simulink model "solar_grid_powered_EV_Battery_Charging_station"  (R2020a)
settings: Solver=VariableStepAuto  StartTime=0.0  StopTime=1  RelTol=1e-3
undefined symbols (not defined in the file): Ion, Lithium
libraries: powerlib x68, simulink x10, powerlib_meascontrol x4, electricdrivelib x1, re_lib x1
(part 1 of 2)
settings Model: Creator=sunil  LastModifiedBy=sunil

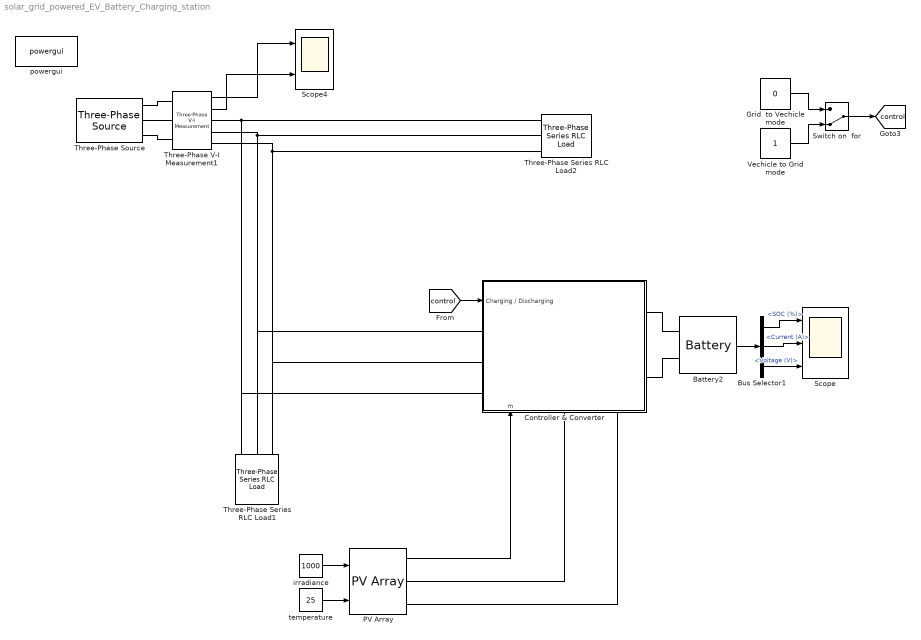
== system solar_grid_powered_EV_Battery_Charging_station ==
  Battery2 : electricdrivelib/Extra Sources/Battery  BatType=Lithium-Ion  ShowTempParam=off  ThermalPreset=no  ShowAgeParam=off  NomV=250  NomQ=300  SOC=80  Batt_Tr=30  PresetModel=on  MaxQ=300  MinV=187.5  FullV=290.9968  Dis_rate=130.4348  R=0.0083333  Normal_OP=271.3043  expZone="[270.0965      14.73913]"  current=[6.5 13 32.5]  Units=Time  Tci=20  NomT=20  T2=-30  MaxQ2=4.8  FullV2=7.1  Normal_OP2=5.655  expZone2="[6.58           1]"  Rca=0.6  ti=2000  Dp=0  Neq0=0  Tsim=1e6  Ta1=25  Qeol=5.4*0.9  Reol=0.013333*1.2  Char_age=[2.3478, 3]  Dis_age=[2.3478, 10]  N1=1500  N2=10500  N3=1000  N4=1400  Ta2=45  N5=950
  Bus Selector1 : BusSelector  OutputSignals=SOC (%),Current (A),Voltage (V)
  Controller & Converter : Subsystem
      settings: PortSchema="{\"entries\":[{\"content\":{\"sides\":[{\"content\":{\"connectorIds\":[\"In1\",\"LConn1\",\"LConn2\",\"LConn3\"]},\"type\":\"ConnectorPlacement.EquallySpacedRectSide\",\"uuid\":\"3304ff68-ecae-43f2-8867-5e121d5d8c98\"},{\"content\":{\"connectorIds\":[\"RConn1\",\"RConn2\"],\"side\":\"RIGHT\"},\"type\":\"ConnectorPlacement.EquallySpacedRectSide\",\"uuid\":\"3bd92547-fde4-4d16-9531-59e3d4d1a2fd\"},{\"content\":{\"connectorIds\":[],\"side\":\"TOP\"},\"type\":\"ConnectorPlacement.EquallySpacedRectSide\",\"uuid\":\"a99ca367-b74d-41f6-b4fc-d39809732728\"},{\"content\":{\"connectorIds\":[\"In2\",\"RConn3\",\"RConn4\"],\"side\":\"BOTTOM\"},\"type\":\"ConnectorPlacement.EquallySpacedRectSide\",\"uuid\":\"df3368a7-37c5-4fdd-8e4a-104a2c6a0ba1\"}]},\"type\":\"ConnectorPlacement.EquallySpacedConnector\",\"uuid\":\"9d0b0e84-d3bf-47a7-98c1-fe37fca38536\"}],\"packageUris\":[\"http://schema.mathworks.com/mf0/Connector/19700101\"],\"version\":\"1.0\"}"
  Grid  to Vechicle mode : Constant  Value=0  VectorParams1D=off  SampleTime=-1
  PV Array : re_lib/Solar/PV Array  Npar=10  Nser=7  PlotType=array @ 25 deg.C & specified irradiances  S_vec="[ 1000  500  100 ]"  Temp_C_vec="[ 45 25  ]"  ModuleName=User-defined  PlotWhenSelected=off  Pm=390.173  Ncell=72  Voc=48.85  Isc=10  Vm=40.1  Im=9.73  beta_Voc_pc=-0.37  alpha_Isc_pc=0.05  beta_Voc=-0.18075  alpha_Isc=0.005  IL=10.1848  I0=4.7391e-10  nI=1.1101  Rsh=3123.3273  Rs=0.27721  RobustModel=off  RobustCellTemperature=25  BAL=on  Tc=1e-6  Tfilter=5e-5
  Scope : Scope  NumInputPorts=3
  Scope4 : Scope  NumInputPorts=2
  "Switch on  for " : ManualSwitch  CurrentSetting=0
  Three-Phase Series RLC Load1 : powerlib/Elements/Three-Phase Series RLC Load  LConnTagsString=A|B|C  Configuration=Y (grounded)  NominalVoltage=415  Vabc=[1e3 1e3 1e3]  Vabcp=[1e3 1e3 1e3]  NominalFrequency=50  UnbalancedPower=off  ActivePower=1e3  InductivePower=0  CapacitivePower=0  Pabc=[10e3 9e3 11e3]  QLabc=[100 90 110]  QCabc=[100 90 110]  Pabcp=[10e3 9e3 11e3]  QLabcp=[100 90 110]  QCabcp=[100 90 110]  Measurements=None  LoadType=constant Z
  Three-Phase Series RLC Load2 : powerlib/Elements/Three-Phase Series RLC Load  LConnTagsString=A|B|C  Configuration=Y (grounded)  NominalVoltage=415  Vabc=[1e3 1e3 1e3]  Vabcp=[1e3 1e3 1e3]  NominalFrequency=50  UnbalancedPower=off  ActivePower=1e-3  InductivePower=0  CapacitivePower=0  Pabc=[10e3 9e3 11e3]  QLabc=[100 90 110]  QCabc=[100 90 110]  Pabcp=[10e3 9e3 11e3]  QLabcp=[100 90 110]  QCabcp=[100 90 110]  Measurements=None  LoadType=constant Z
  Three-Phase V-I Measurement1 : powerlib/Measurements/Three-Phase V-I Measurement  VoltageMeasurement=phase-to-phase  SetLabelV=off  LabelV=Vabc  Vpu=off  VpuLL=off  CurrentMeasurement=yes  SetLabelI=off  LabelI=Iabc  Ipu=off  Pbase=100e6  Vbase=500e3  OutputType=Complex  PhasorSimulation=off  PSBequivalent=0
  Three-Phase Source : powerlib/Electrical Sources/Three-Phase Source  InternalConnection=Yg  VoltagePhases=off  Voltage=415  PhaseAngle=0  Voltage_phases=[25e3 25e3 25e3]/sqrt(3)  PhaseAngles_phases=[0 -120 +120]  Frequency=50  NonIdealSource=on  SpecifyImpedance=off  Resistance=1e-6  Inductance=1e-6  ShortCircuitLevel=100e6  BaseVoltage=415  XRratio=7  BusType=swing  Pref=10e3  Qref=0  Prefabc=[10e3, 10e3, 10e3]  Qrefabc=[0, 0, 0]  Qmin=-inf  Qmax=inf
  Vechicle to Grid mode : Constant  VectorParams1D=off  SampleTime=-1
  irradiance : Constant  Value=1000
  powergui : powerlib/powergui  Priority=1  SimulationMode=Discrete  SampleTime=5e-6  frequency=60  Iterations=50  frequencyindice=0  Pbase=100e6  ErrMax=1e-4  UnitsV=kV  UnitsW=MW  buscounter=0  FunctionMessages=off  echomessages=off  EnableUseOfTLC=off  CurrentSourceSwitches=off  DisableSnubberDevices=off  DisableRonSwitches=off  DisableVfSwitches=off  DisplayEquations=off  AutomaticDiscreteSolvers=off  SolverType=Tustin/Backward Euler (TBE)  Interpol=off  ExternalGateDelay=off  methode=off  Ts=100  x0status=blocks  SPID=on  SwTol=0  HookPort=off  NonlinearTolerance=1e-4  nMaxIteration=100  ContinueOnMaxIteration=off  RestoreLinks=warning  ResistiveCurrentMeasurement=off  Frange=[0:2:500]  Ylog=off  Xlog=on  ShowGrid=off  save=off  variable=ZData  structure=0  ZoomFFT=off  StartTime=0.0  cycles=1  DisplayStyle=1  fundamental=60  FreqAxis=off  MaxFrequency=1000  frequencyindicesteady=1  RmsSteady=1  display=off
  temperature : Constant  Value=25
  tag scope: control=global
  wires:
  Bus Selector1/2 -> Scope/2  "<Current (A)>"
  Grid  to Vechicle mode/1 -> "Switch on  for "/1
  [control] -> Controller & Converter/1(Charging / Discharging)
  Bus Selector1/3 -> Scope/3  "<Voltage (V)>"
  Vechicle to Grid mode/1 -> "Switch on  for "/2
  Bus Selector1/1 -> Scope/1  "<SOC (%)>"
  Three-Phase V-I Measurement1/2 -> Scope4/2
  Battery2/1 -> Bus Selector1/1
  temperature/1 -> PV Array/2
  Three-Phase V-I Measurement1/1 -> Scope4/1
  "Switch on  for "/1 -> [control]
  PV Array/1 -> Controller & Converter/2(m)
  irradiance/1 -> PV Array/1
  connections:
  Three-Phase Series RLC Load2/LConn2 -- Three-Phase Series RLC Load1/LConn2 -- Controller & Converter/LConn1 -- Three-Phase V-I Measurement1/RConn2
  Three-Phase Series RLC Load2/LConn3 -- Three-Phase V-I Measurement1/RConn3 -- Three-Phase Series RLC Load1/LConn3 -- Controller & Converter/LConn2
  Three-Phase Series RLC Load2/LConn1 -- Three-Phase Series RLC Load1/LConn1 -- Controller & Converter/LConn3 -- Three-Phase V-I Measurement1/RConn1
  Battery2/LConn1 -- Controller & Converter/RConn1
  Three-Phase V-I Measurement1/LConn3 -- Three-Phase Source/RConn3
  PV Array/RConn2 -- Controller & Converter/RConn4
  Three-Phase V-I Measurement1/LConn2 -- Three-Phase Source/RConn2
  Battery2/LConn2 -- Controller & Converter/RConn2
  Three-Phase V-I Measurement1/LConn1 -- Three-Phase Source/RConn1
  PV Array/RConn1 -- Controller & Converter/RConn3

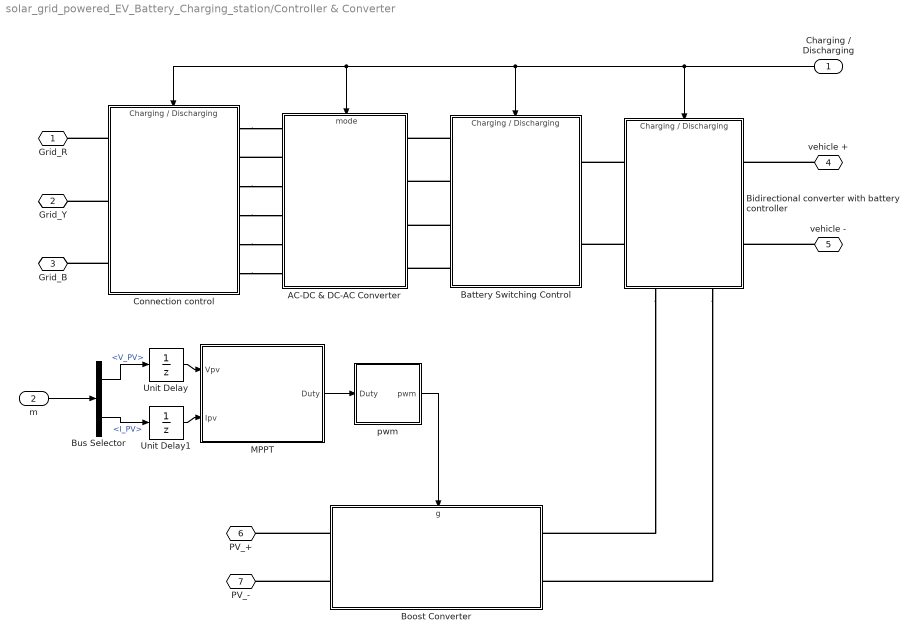
== system solar_grid_powered_EV_Battery_Charging_station/Controller & Converter ==
  Charging / Discharging : Inport
  m : Inport  Port=2
  AC-DC & DC-AC Converter : Subsystem
      settings: PortSchema="{\"entries\":[{\"content\":{\"sides\":[{\"content\":{\"connectorIds\":[\"LConn1\",\"LConn2\",\"LConn3\",\"LConn4\",\"LConn5\",\"LConn6\"]},\"type\":\"ConnectorPlacement.EquallySpacedRectSide\",\"uuid\":\"fb71d267-2bb0-4139-94a5-dc54601bb02f\"},{\"content\":{\"connectorIds\":[\"RConn1\",\"RConn2\",\"RConn3\",\"RConn4\"],\"side\":\"RIGHT\"},\"type\":\"ConnectorPlacement.EquallySpacedRectSide\",\"uuid\":\"de844200-b1ec-408d-a180-7fb4681b7df4\"},{\"content\":{\"connectorIds\":[\"In1\"],\"side\":\"TOP\"},\"type\":\"ConnectorPlacement.EquallySpacedRectSide\",\"uuid\":\"9cac342e-4efb-4690-aa53-18569bafd674\"}]},\"type\":\"ConnectorPlacement.EquallySpacedConnector\",\"uuid\":\"f9655260-9e6f-4e0e-a67b-e2fec888fb30\"}],\"packageUris\":[\"http://schema.mathworks.com/mf0/Connector/19700101\"],\"version\":\"1.0\"}"
  Battery Switching Control : Subsystem
      settings: PortSchema="{\"entries\":[{\"content\":{\"sides\":[{\"content\":{\"connectorIds\":[\"LConn1\",\"LConn2\",\"LConn3\",\"LConn4\"]},\"type\":\"ConnectorPlacement.EquallySpacedRectSide\",\"uuid\":\"d80df2a9-ec6b-4c90-bb66-bcdaf5f87525\"},{\"content\":{\"connectorIds\":[\"RConn1\",\"RConn2\"],\"side\":\"RIGHT\"},\"type\":\"ConnectorPlacement.EquallySpacedRectSide\",\"uuid\":\"2e5caa84-3c0f-4e6e-a9f1-36c129bda481\"},{\"content\":{\"connectorIds\":[\"In1\"],\"side\":\"TOP\"},\"type\":\"ConnectorPlacement.EquallySpacedRectSide\",\"uuid\":\"9ad9ed80-d46f-43fc-be26-7456a6f75322\"},{\"content\":{\"connectorIds\":[],\"side\":\"BOTTOM\"},\"type\":\"ConnectorPlacement.EquallySpacedRectSide\",\"uuid\":\"36c54608-1582-475c-a859-dff20a425875\"}]},\"type\":\"ConnectorPlacement.EquallySpacedConnector\",\"uuid\":\"78778afb-b988-47e6-8bc2-703e283fa2d4\"}],\"packageUris\":[\"http://schema.mathworks.com/mf0/Connector/19700101\"],\"version\":\"1.0\"}"
  Bidirectional converter with battery controller : Subsystem
      settings: PortSchema="{\"entries\":[{\"content\":{\"sides\":[{\"content\":{\"connectorIds\":[\"LConn1\",\"LConn2\"]},\"type\":\"ConnectorPlacement.EquallySpacedRectSide\",\"uuid\":\"86880c34-88a1-4209-bf34-ac5a91279ce4\"},{\"content\":{\"connectorIds\":[\"RConn1\",\"RConn2\"],\"side\":\"RIGHT\"},\"type\":\"ConnectorPlacement.EquallySpacedRectSide\",\"uuid\":\"9dcfc645-7c2c-4fe1-9bcb-24debf25abab\"},{\"content\":{\"connectorIds\":[\"In1\"],\"side\":\"TOP\"},\"type\":\"ConnectorPlacement.EquallySpacedRectSide\",\"uuid\":\"a2f7b554-97d3-490c-a983-3514cfd45afe\"},{\"content\":{\"connectorIds\":[\"RConn3\",\"RConn4\"],\"side\":\"BOTTOM\"},\"type\":\"ConnectorPlacement.EquallySpacedRectSide\",\"uuid\":\"9f51b392-4a7b-4452-b01e-9bc26600887f\"}]},\"type\":\"ConnectorPlacement.EquallySpacedConnector\",\"uuid\":\"53695bd3-452d-4933-bbd5-5b98019d2721\"}],\"packageUris\":[\"http://schema.mathworks.com/mf0/Connector/19700101\"],\"version\":\"1.0\"}"
  Boost Converter : Subsystem
      settings: PortSchema="{\"entries\":[{\"content\":{\"sides\":[{\"content\":{\"connectorIds\":[\"LConn1\",\"LConn2\"]},\"type\":\"ConnectorPlacement.EquallySpacedRectSide\",\"uuid\":\"ba3df88f-bd8f-4585-9ccf-ee80b9ae1df7\"},{\"content\":{\"connectorIds\":[\"RConn1\",\"RConn2\"],\"side\":\"RIGHT\"},\"type\":\"ConnectorPlacement.EquallySpacedRectSide\",\"uuid\":\"07e3c8e5-cf0e-4606-afd9-e4eed787cba4\"},{\"content\":{\"connectorIds\":[\"In1\"],\"side\":\"TOP\"},\"type\":\"ConnectorPlacement.EquallySpacedRectSide\",\"uuid\":\"0b82548a-ce43-4895-b683-aaa03795dd24\"}]},\"type\":\"ConnectorPlacement.EquallySpacedConnector\",\"uuid\":\"1dcff1c7-df30-47a9-a5da-6bd033c00133\"}],\"packageUris\":[\"http://schema.mathworks.com/mf0/Connector/19700101\"],\"version\":\"1.0\"}"
  Bus Selector : BusSelector  OutputSignals=V_PV,I_PV
  Connection control : Subsystem
      settings: PortSchema="{\"entries\":[{\"content\":{\"sides\":[{\"content\":{\"connectorIds\":[\"LConn1\",\"LConn2\",\"LConn3\"]},\"type\":\"ConnectorPlacement.EquallySpacedRectSide\",\"uuid\":\"4b804f5e-ccd8-48e4-9dd4-f3e4f4f04b31\"},{\"content\":{\"connectorIds\":[\"RConn1\",\"RConn2\",\"RConn3\",\"RConn4\",\"RConn5\",\"RConn6\"],\"side\":\"RIGHT\"},\"type\":\"ConnectorPlacement.EquallySpacedRectSide\",\"uuid\":\"f88efa6c-9e5b-45b8-93e8-1425e80d8a81\"},{\"content\":{\"connectorIds\":[\"In1\"],\"side\":\"TOP\"},\"type\":\"ConnectorPlacement.EquallySpacedRectSide\",\"uuid\":\"34942438-89d1-493a-a64f-7ff1173d7d06\"}]},\"type\":\"ConnectorPlacement.EquallySpacedConnector\",\"uuid\":\"62c4ca2c-a19a-421e-ab33-e75936f0a9d2\"}],\"packageUris\":[\"http://schema.mathworks.com/mf0/Connector/19700101\"],\"version\":\"1.0\"}"
  MPPT : Subsystem
  Unit Delay : UnitDelay  SampleTime=1e-4  HasFrameUpgradeWarning=on
  Unit Delay1 : UnitDelay  SampleTime=1e-4  HasFrameUpgradeWarning=on
  pwm : Subsystem
  Grid_R : PMIOPort  Side=Left
  Grid_Y : PMIOPort  Port=2  Side=Left
  Grid_B : PMIOPort  Port=3  Side=Left
  vehicle + : PMIOPort  Port=4  Side=Right
  vehicle - : PMIOPort  Port=5  Side=Right
  PV_+ : PMIOPort  Port=6  Side=Right
  PV_- : PMIOPort  Port=7  Side=Right
  wires:
  Charging / Discharging/1 -> Battery Switching Control/1(Charging / Discharging), AC-DC & DC-AC Converter/1(mode), Connection control/1(Charging / Discharging), Bidirectional converter with battery controller/1(Charging / Discharging)
  Bus Selector/1 -> Unit Delay/1  "<V_PV>"
  Unit Delay1/1 -> MPPT/2(Ipv)
  MPPT/1(Duty) -> pwm/1(Duty)
  Bus Selector/2 -> Unit Delay1/1  "<I_PV>"
  Unit Delay/1 -> MPPT/1(Vpv)
  pwm/1(pwm) -> Boost Converter/1(g)
  m/1 -> Bus Selector/1
  connections:
  Connection control/LConn1 -- Grid_R/RConn1
  Connection control/LConn2 -- Grid_Y/RConn1
  Connection control/LConn3 -- Grid_B/RConn1
  AC-DC & DC-AC Converter/LConn2 -- Connection control/RConn2
  Connection control/RConn1 -- AC-DC & DC-AC Converter/LConn1
  Connection control/RConn3 -- AC-DC & DC-AC Converter/LConn3
  Connection control/RConn4 -- AC-DC & DC-AC Converter/LConn4
  Connection control/RConn5 -- AC-DC & DC-AC Converter/LConn5
  Connection control/RConn6 -- AC-DC & DC-AC Converter/LConn6
  vehicle +/RConn1 -- Bidirectional converter with battery controller/RConn1
  vehicle -/RConn1 -- Bidirectional converter with battery controller/RConn2
  Bidirectional converter with battery controller/LConn1 -- Battery Switching Control/RConn1
  Bidirectional converter with battery controller/LConn2 -- Battery Switching Control/RConn2
  Battery Switching Control/LConn1 -- AC-DC & DC-AC Converter/RConn1
  Battery Switching Control/LConn2 -- AC-DC & DC-AC Converter/RConn2
  Battery Switching Control/LConn3 -- AC-DC & DC-AC Converter/RConn3
  Battery Switching Control/LConn4 -- AC-DC & DC-AC Converter/RConn4
  Boost Converter/LConn1 -- PV_+/RConn1
  Boost Converter/LConn2 -- PV_-/RConn1
  Bidirectional converter with battery controller/RConn3 -- Boost Converter/RConn1
  Bidirectional converter with battery controller/RConn4 -- Boost Converter/RConn2

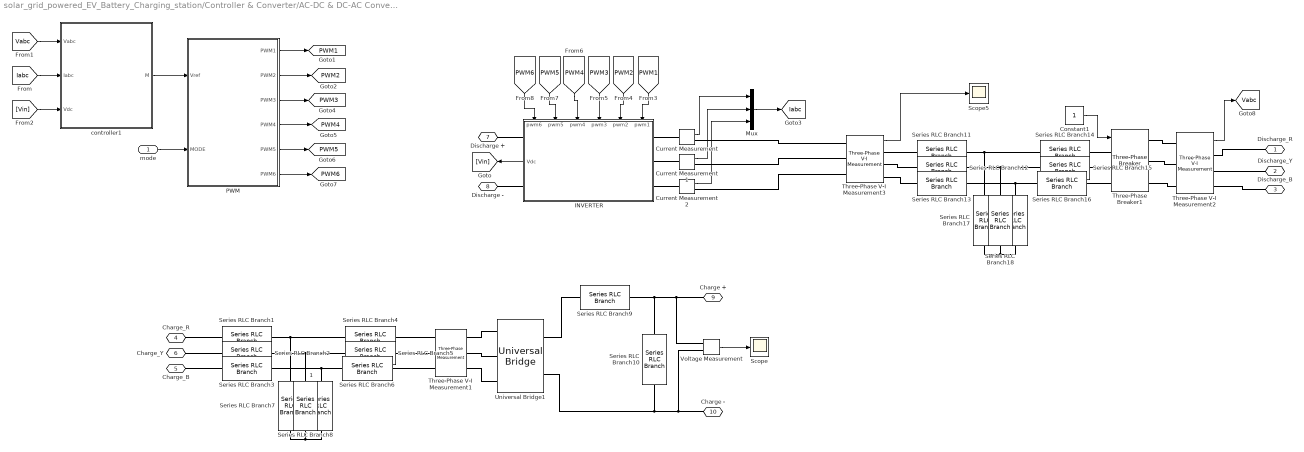
== system solar_grid_powered_EV_Battery_Charging_station/Controller & Converter/AC-DC & DC-AC Converter ==
  mode : Inport
  " " : powerlib/Elements/Series RLC Branch  LConnTagsString=__new0  RConnTagsString=__new0  BranchType=C  Resistance=1  Inductance=500e-6  SetiL0=off  InitialCurrent=0  Capacitance=100e-6  Setx0=off  InitialVoltage=0  Measurements=None
  " 1" : powerlib/Elements/Series RLC Branch  LConnTagsString=__new0  RConnTagsString=__new0  BranchType=C  Resistance=1  Inductance=500e-6  SetiL0=off  InitialCurrent=0  Capacitance=100e-6  Setx0=off  InitialVoltage=0  Measurements=None
  Constant1 : Constant
  Current Measurement : powerlib/Measurements/Current Measurement  PhasorSimulation=off  OutputType=Complex  PSBequivalent=0
  Current Measurement1 : powerlib/Measurements/Current Measurement  PhasorSimulation=off  OutputType=Complex  PSBequivalent=0
  Current Measurement2 : powerlib/Measurements/Current Measurement  PhasorSimulation=off  OutputType=Complex  PSBequivalent=0
  INVERTER : Subsystem
      settings: PortSchema="{\"entries\":[{\"content\":{\"sides\":[{\"content\":{\"connectorIds\":[\"LConn1\",\"Out1\",\"LConn2\"]},\"type\":\"ConnectorPlacement.EquallySpacedRectSide\",\"uuid\":\"c3946ff9-9688-4b39-8168-58c2573ee620\"},{\"content\":{\"connectorIds\":[\"RConn1\",\"RConn2\",\"RConn3\"],\"side\":\"RIGHT\"},\"type\":\"ConnectorPlacement.EquallySpacedRectSide\",\"uuid\":\"a5e23abb-073e-446d-99b2-4b67fe8ba86f\"},{\"content\":{\"connectorIds\":[\"In1\",\"In2\",\"In3\",\"In4\",\"In5\",\"In6\"],\"side\":\"TOP\"},\"type\":\"ConnectorPlacement.EquallySpacedRectSide\",\"uuid\":\"619d3410-10ed-4be1-83e0-3a782e5fb67e\"},{\"content\":{\"connectorIds\":[],\"side\":\"BOTTOM\"},\"type\":\"ConnectorPlacement.EquallySpacedRectSide\",\"uuid\":\"5460b93f-0e8e-403e-90d4-5441007e8d92\"}]},\"type\":\"ConnectorPlacement.EquallySpacedConnector\",\"uuid\":\"e5ca039e-511e-411b-beec-5bfaa270a6f6\"}],\"packageUris\":[\"http://schema.mathworks.com/mf0/Connector/19700101\"],\"version\":\"1.0\"}"
  Mux : Mux  Inputs=3
  PWM : Subsystem
  Scope : Scope
  Scope5 : Scope
  Series RLC Branch{1..6,11..16} (12 alike) : powerlib/Elements/Series RLC Branch  LConnTagsString=__new0  RConnTagsString=__new0  BranchType=L  Resistance=1  Inductance=2000e-6  SetiL0=off  InitialCurrent=0  Capacitance=1e-6  Setx0=off  InitialVoltage=0  Measurements=None
  Series RLC Branch10 : powerlib/Elements/Series RLC Branch  LConnTagsString=__new0  RConnTagsString=__new0  BranchType=C  Resistance=1e-3  Inductance=1e-3  SetiL0=off  InitialCurrent=0  Capacitance=100e-6  Setx0=off  InitialVoltage=0  Measurements=None
  Series RLC Branch{7..8,17..18} (4 alike) : powerlib/Elements/Series RLC Branch  LConnTagsString=__new0  RConnTagsString=__new0  BranchType=C  Resistance=1  Inductance=500e-6  SetiL0=off  InitialCurrent=0  Capacitance=100e-6  Setx0=off  InitialVoltage=0  Measurements=None
  Series RLC Branch9 : powerlib/Elements/Series RLC Branch  LConnTagsString=__new0  RConnTagsString=__new0  BranchType=L  Resistance=1e-3  Inductance=10e-3  SetiL0=off  InitialCurrent=0  Capacitance=500e-6  Setx0=off  InitialVoltage=0  Measurements=None
  Three-Phase V-I Measurement1 : powerlib/Measurements/Three-Phase V-I Measurement  VoltageMeasurement=no  SetLabelV=off  LabelV=Vabc  Vpu=off  VpuLL=off  CurrentMeasurement=no  SetLabelI=off  LabelI=Iabc  Ipu=off  Pbase=100e6  Vbase=500e3  OutputType=Complex  PhasorSimulation=off  PSBequivalent=0
  Three-Phase V-I Measurement2 : powerlib/Measurements/Three-Phase V-I Measurement  VoltageMeasurement=phase-to-phase  SetLabelV=off  LabelV=Vabc  Vpu=off  VpuLL=off  CurrentMeasurement=no  SetLabelI=off  LabelI=Iabc  Ipu=off  Pbase=100e6  Vbase=500e3  OutputType=Complex  PhasorSimulation=off  PSBequivalent=0
  Three-Phase V-I Measurement3 : powerlib/Measurements/Three-Phase V-I Measurement  VoltageMeasurement=phase-to-phase  SetLabelV=off  LabelV=Vabc  Vpu=off  VpuLL=off  CurrentMeasurement=no  SetLabelI=off  LabelI=Iabc  Ipu=off  Pbase=100e6  Vbase=500e3  OutputType=Complex  PhasorSimulation=off  PSBequivalent=0
  Three-Phase Breaker1 : powerlib/Elements/Three-Phase Breaker  InitialState=closed  SwitchA=on  SwitchB=on  SwitchC=on  SwitchTimes="[1/60  5/60]"  External=on  BreakerResistance=0.01  SnubberResistance=1e6  SnubberCapacitance=inf  Measurements=None
  Universal Bridge1 : powerlib/Power Electronics/Universal Bridge  Arms=3  SnubberResistance=1e5  SnubberCapacitance=inf  Device=Diodes  Ron=1e-3  Lon=0  ForwardVoltages="[  0  0  ]"  ForwardVoltage=0  GTOparameters=[ 10e-6 , 20e-6 ]  IGBTparameters=[ 1e-6 , 2e-6 ]  Measurements=None  Measurements_2=None  converterType=Rectifier
  Voltage Measurement : powerlib/Measurements/Voltage Measurement  PhasorSimulation=off  OutputType=Complex  PSBequivalent=0
  controller1 : Subsystem
  Discharge_R : PMIOPort  Side=Left
  Discharge_Y : PMIOPort  Port=2  Side=Left
  Discharge_B : PMIOPort  Port=3  Side=Left
  Charge_R : PMIOPort  Port=4  Side=Left
  Charge_B : PMIOPort  Port=5  Side=Left
  Charge_Y : PMIOPort  Port=6  Side=Left
  Discharge + : PMIOPort  Port=7  Side=Right
  Discharge - : PMIOPort  Port=8  Side=Right
  Charge + : PMIOPort  Port=9  Side=Right
  Charge - : PMIOPort  Port=10  Side=Right
  tag scope: Iabc=global, PWM1=global, PWM2=global, PWM3=global, PWM4=global, PWM5=global, PWM6=global, Vabc=global
  wires:
  Voltage Measurement/1 -> Scope/1
  [Vabc] -> controller1/1(Vabc)
  [Vin] -> controller1/3(Vdc)
  PWM/1(PWM1) -> [PWM1]
  PWM/2(PWM2) -> [PWM2]
  [Iabc] -> controller1/2(Iabc)
  controller1/1(M) -> PWM/1(Vref)
  PWM/5(PWM5) -> [PWM5]
  PWM/6(PWM6) -> [PWM6]
  PWM/4(PWM4) -> [PWM4]
  PWM/3(PWM3) -> [PWM3]
  [PWM4] -> INVERTER/3(pwm4)
  [PWM6] -> INVERTER/1(pwm6)
  Current Measurement2/1 -> Mux/3
  [PWM1] -> INVERTER/6(pwm1)
  Current Measurement1/1 -> Mux/2
  [PWM3] -> INVERTER/4(pwm3)
  [PWM5] -> INVERTER/2(pwm5)
  [PWM2] -> INVERTER/5(pwm2)
  Mux/1 -> [Iabc]
  Three-Phase V-I Measurement3/1 -> Scope5/1
  Current Measurement/1 -> Mux/1
  INVERTER/1(Vdc) -> [Vin]
  Three-Phase V-I Measurement2/1 -> [Vabc]
  Constant1/1 -> Three-Phase Breaker1/1
  mode/1 -> PWM/2(MODE)
  connections:
  Series RLC Branch10/RConn1 -- Series RLC Branch9/LConn1 -- Charge +/RConn1 -- Voltage Measurement/LConn1
  Series RLC Branch10/LConn1 -- Voltage Measurement/LConn2 -- Charge -/RConn1 -- Universal Bridge1/RConn2
  Series RLC Branch9/RConn1 -- Universal Bridge1/RConn1
  Three-Phase V-I Measurement1/LConn1 -- Universal Bridge1/LConn1
  Universal Bridge1/LConn2 -- Three-Phase V-I Measurement1/LConn2
  Universal Bridge1/LConn3 -- Three-Phase V-I Measurement1/LConn3
  Series RLC Branch17/LConn1 -- Series RLC Branch11/RConn1 -- Series RLC Branch14/LConn1
  " "/LConn1 -- Series RLC Branch16/LConn1 -- Series RLC Branch13/RConn1
  Series RLC Branch18/LConn1 -- Series RLC Branch15/LConn1 -- Series RLC Branch12/RConn1
  Series RLC Branch12/LConn1 -- Three-Phase V-I Measurement3/RConn2
  Current Measurement1/LConn1 -- INVERTER/RConn2
  Current Measurement/LConn1 -- INVERTER/RConn1
  Three-Phase Breaker1/LConn3 -- Series RLC Branch16/RConn1
  Three-Phase Breaker1/LConn1 -- Series RLC Branch14/RConn1
  Three-Phase V-I Measurement3/LConn2 -- Current Measurement1/RConn1
  Three-Phase Breaker1/LConn2 -- Series RLC Branch15/RConn1
  Three-Phase V-I Measurement3/LConn3 -- Current Measurement2/RConn1
  Series RLC Branch11/LConn1 -- Three-Phase V-I Measurement3/RConn1
  Series RLC Branch13/LConn1 -- Three-Phase V-I Measurement3/RConn3
  Three-Phase V-I Measurement3/LConn1 -- Current Measurement/RConn1
  Current Measurement2/LConn1 -- INVERTER/RConn3
  Discharge -/RConn1 -- INVERTER/LConn2
  Discharge +/RConn1 -- INVERTER/LConn1
  Series RLC Branch18/RConn1 -- Series RLC Branch17/RConn1 -- " "/RConn1
  Series RLC Branch8/LConn1 -- Series RLC Branch5/LConn1 -- Series RLC Branch2/RConn1
  Series RLC Branch8/RConn1 -- Series RLC Branch7/RConn1 -- " 1"/RConn1
  " 1"/LConn1 -- Series RLC Branch6/LConn1 -- Series RLC Branch3/RConn1
  Series RLC Branch4/RConn1 -- Three-Phase V-I Measurement1/RConn1
  Three-Phase V-I Measurement1/RConn2 -- Series RLC Branch5/RConn1
  Three-Phase V-I Measurement1/RConn3 -- Series RLC Branch6/RConn1
  Series RLC Branch7/LConn1 -- Series RLC Branch4/LConn1 -- Series RLC Branch1/RConn1
  Charge_Y/RConn1 -- Series RLC Branch2/LConn1
  Charge_R/RConn1 -- Series RLC Branch1/LConn1
  Charge_B/RConn1 -- Series RLC Branch3/LConn1
  Three-Phase V-I Measurement2/LConn2 -- Three-Phase Breaker1/RConn2
  Three-Phase V-I Measurement2/LConn1 -- Three-Phase Breaker1/RConn1
  Three-Phase V-I Measurement2/LConn3 -- Three-Phase Breaker1/RConn3
  Three-Phase V-I Measurement2/RConn1 -- Discharge_R/RConn1
  Three-Phase V-I Measurement2/RConn2 -- Discharge_Y/RConn1
  Discharge_B/RConn1 -- Three-Phase V-I Measurement2/RConn3

== system solar_grid_powered_EV_Battery_Charging_station/Controller & Converter/Battery Switching Control ==
  Charging / Discharging : Inport
  Ideal Switch{,1..3} (4 alike) : powerlib/Power Electronics/Ideal Switch  Ron=0.001  Lon=0  IC=0  Rs=1e5  Cs=inf  Measurements=off
  NOT : Logic  Operator=NOT  IconShape=distinctive  AllPortsSameDT=off  OutDataTypeStr=boolean
  Discharge + : PMIOPort  Side=Left
  Discharge - : PMIOPort  Port=2  Side=Left
  Charge + : PMIOPort  Port=3  Side=Left
  Charge - : PMIOPort  Port=4  Side=Left
  Converter + : PMIOPort  Port=5  Side=Right
  Converter - : PMIOPort  Port=6  Side=Right
  wires:
  Charging / Discharging/1 -> Ideal Switch/1, NOT/1, Ideal Switch1/1
  NOT/1 -> Ideal Switch3/1, Ideal Switch2/1
  connections:
  Ideal Switch1/LConn1 -- Ideal Switch3/LConn1 -- Converter -/RConn1
  Ideal Switch/LConn1 -- Ideal Switch2/LConn1 -- Converter +/RConn1
  Ideal Switch/RConn1 -- Discharge +/RConn1
  Ideal Switch1/RConn1 -- Discharge -/RConn1
  Ideal Switch2/RConn1 -- Charge +/RConn1
  Ideal Switch3/RConn1 -- Charge -/RConn1

== system solar_grid_powered_EV_Battery_Charging_station/Controller & Converter/Bidirectional converter with battery controller ==
  Charging / Discharging : Inport
  Bi-directional Converter : Subsystem
      settings: PortSchema="{\"entries\":[{\"content\":{\"sides\":[{\"content\":{\"connectorIds\":[\"LConn1\",\"LConn2\"]},\"type\":\"ConnectorPlacement.EquallySpacedRectSide\",\"uuid\":\"6185904c-6dfb-4564-aa03-1b7bee9041cf\"},{\"content\":{\"connectorIds\":[\"RConn1\",\"RConn2\"],\"side\":\"RIGHT\"},\"type\":\"ConnectorPlacement.EquallySpacedRectSide\",\"uuid\":\"b77d5c95-3c24-4f78-895a-d4b58bed9bc2\"},{\"content\":{\"connectorIds\":[\"In1\",\"In2\"],\"side\":\"TOP\"},\"type\":\"ConnectorPlacement.EquallySpacedRectSide\",\"uuid\":\"25e41475-f3e5-4c0a-8bdf-1a6173604e77\"},{\"content\":{\"connectorIds\":[],\"side\":\"BOTTOM\"},\"type\":\"ConnectorPlacement.EquallySpacedRectSide\",\"uuid\":\"107dbda6-1f7c-4f0c-ac4f-8f51f9a6b3ae\"}]},\"type\":\"ConnectorPlacement.EquallySpacedConnector\",\"uuid\":\"36757667-4446-4307-8c42-a960e513f0e6\"}],\"packageUris\":[\"http://schema.mathworks.com/mf0/Connector/19700101\"],\"version\":\"1.0\"}"
  controller : Subsystem
      settings: PortSchema="{\"entries\":[{\"content\":{\"sides\":[{\"content\":{\"connectorIds\":[\"In1\",\"In2\",\"In3\"]},\"type\":\"ConnectorPlacement.EquallySpacedRectSide\",\"uuid\":\"b3ccd9fb-ed03-49d3-87f8-7565ee8d1ba8\"},{\"content\":{\"connectorIds\":[\"Out1\",\"Out2\"],\"side\":\"RIGHT\"},\"type\":\"ConnectorPlacement.EquallySpacedRectSide\",\"uuid\":\"c15ee824-c5c9-428d-b80b-68bfa14ee36f\"},{\"content\":{\"connectorIds\":[\"In4\"],\"side\":\"TOP\"},\"type\":\"ConnectorPlacement.EquallySpacedRectSide\",\"uuid\":\"0088a958-a830-4424-88e1-02f84920e46e\"}]},\"type\":\"ConnectorPlacement.EquallySpacedConnector\",\"uuid\":\"ed0e5d7c-dffd-42fc-9728-84b14c62e70f\"}],\"packageUris\":[\"http://schema.mathworks.com/mf0/Connector/19700101\"],\"version\":\"1.0\"}"
  Converter + : PMIOPort  Side=Left
  Converter  - : PMIOPort  Port=2  Side=Left
  Battery + : PMIOPort  Port=3  Side=Right
  Battery - : PMIOPort  Port=4  Side=Right
  PV_out+ : PMIOPort  Port=5  Side=Right
  PV_out_- : PMIOPort  Port=6  Side=Right
  wires:
  Charging / Discharging/1 -> controller/4(CONTROL)
  [Ib] -> controller/2(Ib)
  [Vb] -> controller/3(Vb)
  [Vin] -> controller/1(Vin)
  controller/1(pwm_discharging) -> Bi-directional Converter/2(Discharging)
  controller/2(pwm_charging) -> Bi-directional Converter/1(Charging)
  connections:
  Converter  -/RConn1 -- Bi-directional Converter/LConn2 -- PV_out_-/RConn1
  Converter +/RConn1 -- PV_out+/RConn1 -- Bi-directional Converter/LConn1
  Battery +/RConn1 -- Bi-directional Converter/RConn1
  Battery -/RConn1 -- Bi-directional Converter/RConn2

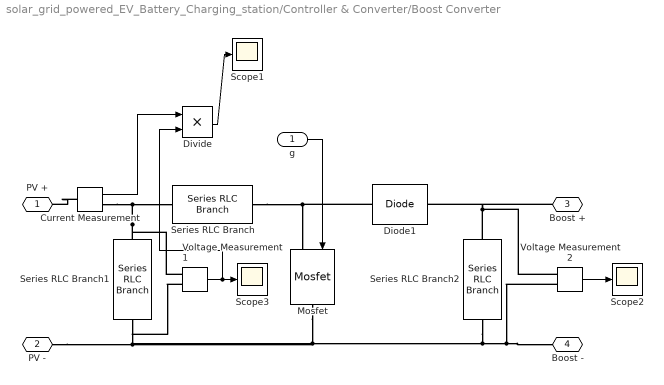
== system solar_grid_powered_EV_Battery_Charging_station/Controller & Converter/Boost Converter ==
  g : Inport
  Current Measurement : powerlib/Measurements/Current Measurement  PhasorSimulation=off  OutputType=Complex  PSBequivalent=0
  Diode1 : powerlib/Power Electronics/Diode  Ron=0.001  Lon=0  Vf=0.8  IC=0  UseSnubber=off  Rs=500  Cs=250e-9  Measurements=off
  Divide : Product  Inputs=**
  Mosfet : powerlib/Power Electronics/Mosfet  Ron=0.1  Lon=0  Rd=0.01  Vfd=0  IC=0  Rs=1e5  Cs=inf  Measurements=off
  Scope1 : Scope
  Scope2 : Scope
  Scope3 : Scope
  Series RLC Branch : powerlib/Elements/Series RLC Branch  LConnTagsString=__new0  RConnTagsString=__new0  BranchType=L  Resistance=1  Inductance=540e-3  SetiL0=off  InitialCurrent=0  Capacitance=1e-6  Setx0=off  InitialVoltage=0  Measurements=None
  Series RLC Branch1 : powerlib/Elements/Series RLC Branch  LConnTagsString=__new0  RConnTagsString=__new0  BranchType=RC  Resistance=.0001  Inductance=1e-3  SetiL0=off  InitialCurrent=0  Capacitance=100e-6  Setx0=off  InitialVoltage=0  Measurements=None
  Series RLC Branch2 : powerlib/Elements/Series RLC Branch  LConnTagsString=__new0  RConnTagsString=__new0  BranchType=C  Resistance=1  Inductance=1e-3  SetiL0=off  InitialCurrent=0  Capacitance=8750e-6  Setx0=off  InitialVoltage=0  Measurements=None
  Voltage Measurement1 : powerlib/Measurements/Voltage Measurement  PhasorSimulation=off  OutputType=Complex  PSBequivalent=0
  Voltage Measurement2 : powerlib/Measurements/Voltage Measurement  PhasorSimulation=off  OutputType=Complex  PSBequivalent=0
  PV + : PMIOPort  Side=Left
  PV - : PMIOPort  Port=2  Side=Left
  Boost + : PMIOPort  Port=3  Side=Right
  Boost - : PMIOPort  Port=4  Side=Right
  wires:
  Voltage Measurement1/1 -> Divide/2, Scope3/1
  g/1 -> Mosfet/1
  Current Measurement/1 -> Divide/1
  Divide/1 -> Scope1/1
  Voltage Measurement2/1 -> Scope2/1
  connections:
  Diode1/LConn1 -- Series RLC Branch/RConn1 -- Mosfet/LConn1
  Voltage Measurement1/LConn1 -- Series RLC Branch1/LConn1 -- Series RLC Branch/LConn1 -- Current Measurement/RConn1
  Series RLC Branch2/LConn1 -- Boost +/RConn1 -- Diode1/RConn1 -- Voltage Measurement2/LConn1
  Series RLC Branch2/RConn1 -- Mosfet/RConn1 -- Series RLC Branch1/RConn1 -- Voltage Measurement1/LConn2 -- PV -/RConn1 -- Voltage Measurement2/LConn2 -- Boost -/RConn1
  Current Measurement/LConn1 -- PV +/RConn1

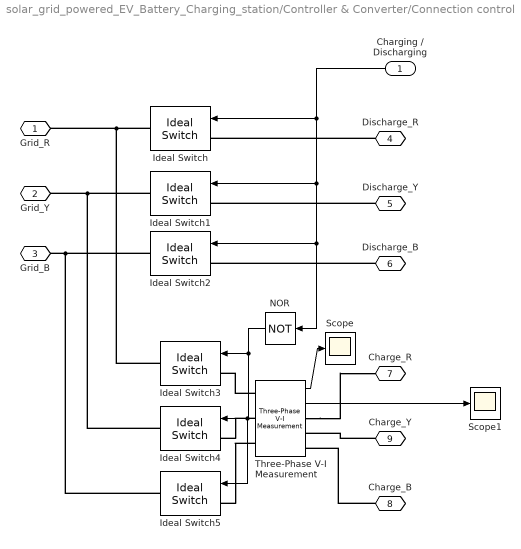
== system solar_grid_powered_EV_Battery_Charging_station/Controller & Converter/Connection control ==
  Charging / Discharging : Inport
  Ideal Switch{,1..5} (6 alike) : powerlib/Power Electronics/Ideal Switch  Ron=0.001  Lon=0  IC=0  Rs=1e5  Cs=inf  Measurements=off
  NOR : Logic  Operator=NOT  IconShape=distinctive  AllPortsSameDT=off  OutDataTypeStr=boolean
  Scope : Scope
  Scope1 : Scope
  Three-Phase V-I Measurement : powerlib/Measurements/Three-Phase V-I Measurement  VoltageMeasurement=phase-to-ground  SetLabelV=off  LabelV=Vabc  Vpu=off  VpuLL=off  CurrentMeasurement=yes  SetLabelI=off  LabelI=Iabc  Ipu=off  Pbase=100e6  Vbase=500e3  OutputType=Complex  PhasorSimulation=off  PSBequivalent=0
  Grid_R : PMIOPort  Side=Left
  Grid_Y : PMIOPort  Port=2  Side=Left
  Grid_B : PMIOPort  Port=3  Side=Left
  Discharge_R : PMIOPort  Port=4  Side=Right
  Discharge_Y : PMIOPort  Port=5  Side=Right
  Discharge_B : PMIOPort  Port=6  Side=Right
  Charge_R : PMIOPort  Port=7  Side=Right
  Charge_B : PMIOPort  Port=8  Side=Right
  Charge_Y : PMIOPort  Port=9  Side=Right
  wires:
  NOR/1 -> Ideal Switch5/1, Ideal Switch4/1, Ideal Switch3/1
  Charging / Discharging/1 -> Ideal Switch/1, Ideal Switch1/1, Ideal Switch2/1, NOR/1
  Three-Phase V-I Measurement/2 -> Scope1/1
  Three-Phase V-I Measurement/1 -> Scope/1
  connections:
  Ideal Switch/RConn1 -- Ideal Switch3/RConn1 -- Grid_R/RConn1
  Discharge_R/RConn1 -- Ideal Switch/LConn1
  Discharge_Y/RConn1 -- Ideal Switch1/LConn1
  Ideal Switch1/RConn1 -- Ideal Switch4/RConn1 -- Grid_Y/RConn1
  Discharge_B/RConn1 -- Ideal Switch2/LConn1
  Ideal Switch2/RConn1 -- Ideal Switch5/RConn1 -- Grid_B/RConn1
  Three-Phase V-I Measurement/LConn1 -- Ideal Switch3/LConn1
  Three-Phase V-I Measurement/LConn2 -- Ideal Switch4/LConn1
  Three-Phase V-I Measurement/LConn3 -- Ideal Switch5/LConn1
  Three-Phase V-I Measurement/RConn1 -- Charge_R/RConn1
  Charge_Y/RConn1 -- Three-Phase V-I Measurement/RConn2
  Charge_B/RConn1 -- Three-Phase V-I Measurement/RConn3

== system solar_grid_powered_EV_Battery_Charging_station/Controller & Converter/MPPT ==
  Vpv : Inport
  Ipv : Inport  Port=2
  P&O_MPPT : MATLAB Function  TreatAsAtomicUnit=on
  Duty : Outport
  wires:
  P&O_MPPT/1(D) -> Duty/1
  Vpv/1 -> P&O_MPPT/1(Vpv)
  Ipv/1 -> P&O_MPPT/2(Ipv)

== system solar_grid_powered_EV_Battery_Charging_station/Controller & Converter/pwm ==
  Duty : Inport
  Relational Operator : RelationalOperator  OutDataTypeStr=boolean  RndMeth=Nearest
  Repeating Sequence : simulink/Sources/Repeating Sequence  rep_seq_t=[0 1/5000]  rep_seq_y=[0 1]
  Scope : Scope
  Scope1 : Scope
  pwm : Outport
  wires:
  Repeating Sequence/1 -> Relational Operator/2, Scope/1
  Relational Operator/1 -> Scope1/1, pwm/1
  Duty/1 -> Relational Operator/1

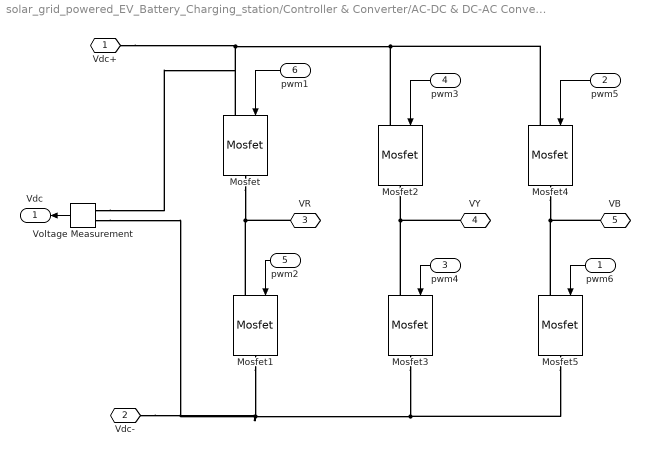
== system solar_grid_powered_EV_Battery_Charging_station/Controller & Converter/AC-DC & DC-AC Converter/INVERTER ==
  pwm6 : Inport
  pwm5 : Inport  Port=2
  pwm4 : Inport  Port=3
  pwm3 : Inport  Port=4
  pwm2 : Inport  Port=5
  pwm1 : Inport  Port=6
  Mosfet{,1..5} (6 alike) : powerlib/Power Electronics/Mosfet  Ron=0.1  Lon=0  Rd=0.01  Vfd=0  IC=0  Rs=1e5  Cs=inf  Measurements=off
  Voltage Measurement : powerlib/Measurements/Voltage Measurement  PhasorSimulation=off  OutputType=Complex  PSBequivalent=0
  Vdc+ : PMIOPort  Side=Left
  Vdc- : PMIOPort  Port=2  Side=Left
  VR : PMIOPort  Port=3  Side=Right
  VY : PMIOPort  Port=4  Side=Right
  VB : PMIOPort  Port=5  Side=Right
  Vdc : Outport
  wires:
  pwm5/1 -> Mosfet4/1
  pwm6/1 -> Mosfet5/1
  pwm1/1 -> Mosfet/1
  pwm2/1 -> Mosfet1/1
  pwm3/1 -> Mosfet2/1
  pwm4/1 -> Mosfet3/1
  Voltage Measurement/1 -> Vdc/1
  connections:
  VR/RConn1 -- Mosfet1/LConn1 -- Mosfet/RConn1
  Mosfet1/RConn1 -- Mosfet3/RConn1 -- Mosfet5/RConn1 -- Vdc-/RConn1 -- Voltage Measurement/LConn2
  VY/RConn1 -- Mosfet2/RConn1 -- Mosfet3/LConn1
  VB/RConn1 -- Mosfet4/RConn1 -- Mosfet5/LConn1
  Vdc+/RConn1 -- Mosfet4/LConn1 -- Mosfet2/LConn1 -- Voltage Measurement/LConn1 -- Mosfet/LConn1

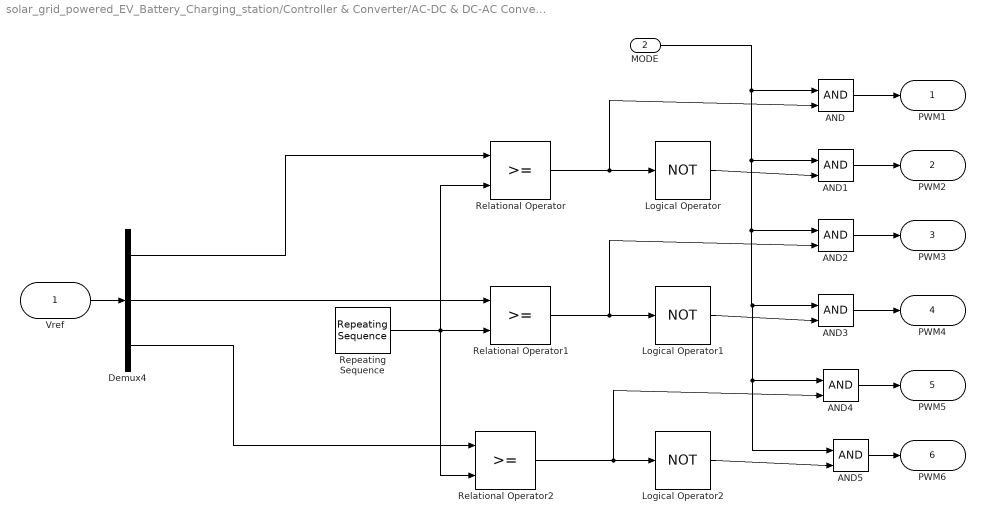
== system solar_grid_powered_EV_Battery_Charging_station/Controller & Converter/AC-DC & DC-AC Converter/PWM ==
  Vref : Inport
  MODE : Inport  Port=2
  AND{,1..5} (6 alike) : Logic  IconShape=distinctive  AllPortsSameDT=off  OutDataTypeStr=boolean
  Demux4 : Demux  Outputs=3
  Logical Operator : Logic  Operator=NOT  AllPortsSameDT=off  OutDataTypeStr=boolean
  Logical Operator1 : Logic  Operator=NOT  AllPortsSameDT=off  OutDataTypeStr=boolean
  Logical Operator2 : Logic  Operator=NOT  AllPortsSameDT=off  OutDataTypeStr=boolean
  Relational Operator : RelationalOperator  OutDataTypeStr=boolean  RndMeth=Nearest
  Relational Operator1 : RelationalOperator  OutDataTypeStr=boolean  RndMeth=Nearest
  Relational Operator2 : RelationalOperator  OutDataTypeStr=boolean  RndMeth=Nearest
  Repeating Sequence : simulink/Sources/Repeating Sequence  rep_seq_t=[0 1/20000 1/10000]  rep_seq_y="[-415  415  -415]"
  PWM1 : Outport
  PWM2 : Outport  Port=2
  PWM3 : Outport  Port=3
  PWM4 : Outport  Port=4
  PWM5 : Outport  Port=5
  PWM6 : Outport  Port=6
  wires:
  Relational Operator1/1 -> AND2/2, Logical Operator1/1
  Relational Operator/1 -> AND/2, Logical Operator/1
  Demux4/1 -> Relational Operator/1
  Demux4/3 -> Relational Operator2/1
  Demux4/2 -> Relational Operator1/1
  Repeating Sequence/1 -> Relational Operator/2, Relational Operator2/2, Relational Operator1/2
  Relational Operator2/1 -> AND4/2, Logical Operator2/1
  Vref/1 -> Demux4/1
  AND/1 -> PWM1/1
  AND1/1 -> PWM2/1
  Logical Operator/1 -> AND1/2
  AND2/1 -> PWM3/1
  AND3/1 -> PWM4/1
  Logical Operator1/1 -> AND3/2
  AND4/1 -> PWM5/1
  Logical Operator2/1 -> AND5/2
  AND5/1 -> PWM6/1
  MODE/1 -> AND5/1, AND4/1, AND3/1, AND2/1, AND1/1, AND/1

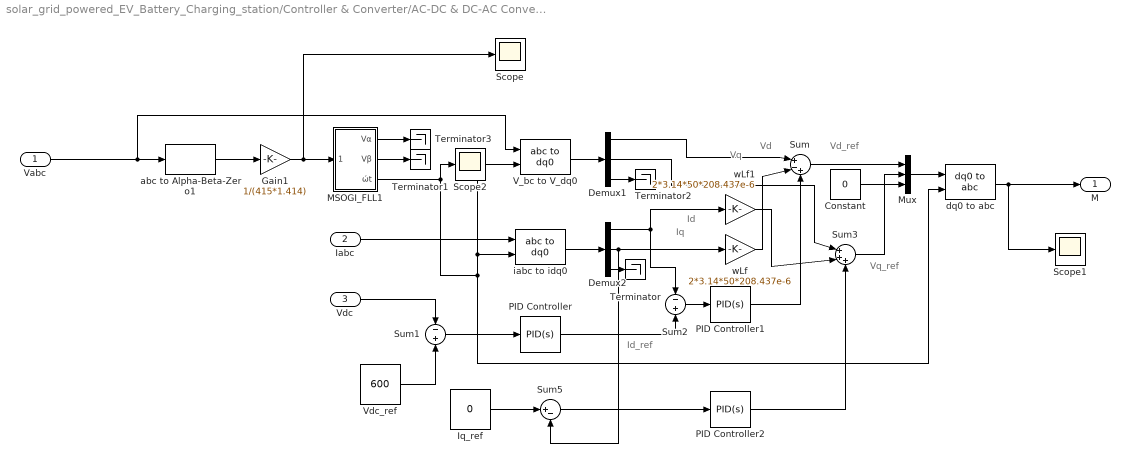
== system solar_grid_powered_EV_Battery_Charging_station/Controller & Converter/AC-DC & DC-AC Converter/controller1 ==
  note: Vd_ref
  note: Id_ref
  note: Id
  note: Vd
  note: Iq
  note: Vq
  note: Vq_ref
  Vabc : Inport
  Iabc : Inport  Port=2
  Vdc : Inport  Port=3
  Constant : Constant  Value=0
  Demux1 : Demux  Outputs=3
  Demux2 : Demux  Outputs=3
  Gain1 : Gain  Gain=1/(415*1.414)
  Iq_ref : Constant  Value=0  VectorParams1D=off  SampleTime=-1
  MSOGI_FLL1 : Subsystem
  Mux : Mux  Inputs=3
  PID Controller : simulink/Continuous/PID Controller  Controller=PID  Form=Parallel  TimeDomain=Continuous-time  UseExternalTs=off  SampleTime=-1  IntegratorMethod=Forward Euler  FilterMethod=Forward Euler  ControllerParametersSource=internal  P=.1  I=1  D=0  UseFilter=on  N=100  TunerSelectOption=Transfer Function Based (PID Tuner App)  InitialConditionSource=internal  InitialConditionForIntegrator=0  InitialConditionForFilter=0  DifferentiatorICPrevScaledInput=0  ExternalReset=none  TrackingMode=off  Kt=1  LimitOutput=off  UpperSaturationLimit=inf  LowerSaturationLimit=-inf  LinearizeAsGain=on  AntiWindupMode=none  Kb=1  POutMin=[]  POutMax=[]  IOutMin=[]  IOutMax=[]  DOutMin=[]  DOutMax=[]  NOutMin=[]  NOutMax=[]  SumOutMin=[]  SumOutMax=[]  SaturationOutMin=[]  SaturationOutMax=[]  PParamMin=[]  PParamMax=[]  IParamMin=[]  IParamMax=[]  DParamMin=[]  DParamMax=[]  NParamMin=[]  NParamMax=[]  KbParamMin=[]  KbParamMax=[]  KtParamMin=[]  KtParamMax=[]  KbOutMin=[]  KbOutMax=[]  KtOutMin=[]  KtOutMax=[]  IntegratorOutMin=[]  IntegratorOutMax=[]  FilterOutMin=[]  FilterOutMax=[]  SumI1OutMin=[]  SumI1OutMax=[]  SumI2OutMin=[]  SumI2OutMax=[]  SumI3OutMin=[]  SumI3OutMax=[]  SumI4OutMin=[]  SumI4OutMax=[]  SumDOutMin=[]  SumDOutMax=[]  DifferentiatorOutMin=[]  DifferentiatorOutMax=[]  FilterDiffOutCoefMin=[]  FilterDiffOutCoefMax=[]  ReciprocalOutMin=[]  ReciprocalOutMax=[]  SumDenOutMin=[]  SumDenOutMax=[]  SumNumOutMin=[]  SumNumOutMax=[]  DivideOutMin=[]  DivideOutMax=[]  UdiffTsProdOutMin=[]  UdiffTsProdOutMax=[]  NTsProdOutMin=[]  NTsProdOutMax=[]  UintegralTsProdOutMin=[]  UintegralTsProdOutMax=[]  UngainTsProdOutMin=[]  UngainTsProdOutMax=[]  IntegratorContinuousStateAttributes=''  IntegratorStateMustResolveToSignalObject=off  IntegratorRTWStateStorageClass=Auto  FilterContinuousStateAttributes=''  FilterStateMustResolveToSignalObject=off  FilterRTWStateStorageClass=Auto  ParallelPVariant=InternalParameters  IdealPVariant=Disabled  IVariant=InternalParameters  DVariant=InternalParameters  IntegratorVariant=Continuous  SatVariant=Disabled  AWVariant=Passthrough  PCopyVariant=Disabled  TRVariant=Disabled  FdbkBlocksVariant=Forward  IdealPFdbkVariant=Disabled  SatFdbkVariant=Disabled  DerivativeFilterVariant=ContFilter  NVariant=InternalParameters  NCopyVariant=Disabled  FilterICVariant=InternalICsFilter  IntegratorICVariant=InternalICs  ExternalResetVariant=Disabled  TRSumVariant=Passthrough  SumFdbkVariant=Disabled  SumVariant=Sum_PID  TsampFilterVariant=InternalTs  TsampNgainVariant=Passthrough  TsampIntegralVariant=Passthrough
  PID Controller1 : simulink/Continuous/PID Controller  Controller=PID  Form=Parallel  TimeDomain=Continuous-time  UseExternalTs=off  SampleTime=-1  IntegratorMethod=Forward Euler  FilterMethod=Forward Euler  ControllerParametersSource=internal  P=.01  I=1  D=0  UseFilter=on  N=100  TunerSelectOption=Transfer Function Based (PID Tuner App)  InitialConditionSource=internal  InitialConditionForIntegrator=0  InitialConditionForFilter=0  DifferentiatorICPrevScaledInput=0  ExternalReset=none  TrackingMode=off  Kt=1  LimitOutput=off  UpperSaturationLimit=inf  LowerSaturationLimit=-inf  LinearizeAsGain=on  AntiWindupMode=none  Kb=1  POutMin=[]  POutMax=[]  IOutMin=[]  IOutMax=[]  DOutMin=[]  DOutMax=[]  NOutMin=[]  NOutMax=[]  SumOutMin=[]  SumOutMax=[]  SaturationOutMin=[]  SaturationOutMax=[]  PParamMin=[]  PParamMax=[]  IParamMin=[]  IParamMax=[]  DParamMin=[]  DParamMax=[]  NParamMin=[]  NParamMax=[]  KbParamMin=[]  KbParamMax=[]  KtParamMin=[]  KtParamMax=[]  KbOutMin=[]  KbOutMax=[]  KtOutMin=[]  KtOutMax=[]  IntegratorOutMin=[]  IntegratorOutMax=[]  FilterOutMin=[]  FilterOutMax=[]  SumI1OutMin=[]  SumI1OutMax=[]  SumI2OutMin=[]  SumI2OutMax=[]  SumI3OutMin=[]  SumI3OutMax=[]  SumI4OutMin=[]  SumI4OutMax=[]  SumDOutMin=[]  SumDOutMax=[]  DifferentiatorOutMin=[]  DifferentiatorOutMax=[]  FilterDiffOutCoefMin=[]  FilterDiffOutCoefMax=[]  ReciprocalOutMin=[]  ReciprocalOutMax=[]  SumDenOutMin=[]  SumDenOutMax=[]  SumNumOutMin=[]  SumNumOutMax=[]  DivideOutMin=[]  DivideOutMax=[]  UdiffTsProdOutMin=[]  UdiffTsProdOutMax=[]  NTsProdOutMin=[]  NTsProdOutMax=[]  UintegralTsProdOutMin=[]  UintegralTsProdOutMax=[]  UngainTsProdOutMin=[]  UngainTsProdOutMax=[]  IntegratorContinuousStateAttributes=''  IntegratorStateMustResolveToSignalObject=off  IntegratorRTWStateStorageClass=Auto  FilterContinuousStateAttributes=''  FilterStateMustResolveToSignalObject=off  FilterRTWStateStorageClass=Auto  ParallelPVariant=InternalParameters  IdealPVariant=Disabled  IVariant=InternalParameters  DVariant=InternalParameters  IntegratorVariant=Continuous  SatVariant=Disabled  AWVariant=Passthrough  PCopyVariant=Disabled  TRVariant=Disabled  FdbkBlocksVariant=Forward  IdealPFdbkVariant=Disabled  SatFdbkVariant=Disabled  DerivativeFilterVariant=ContFilter  NVariant=InternalParameters  NCopyVariant=Disabled  FilterICVariant=InternalICsFilter  IntegratorICVariant=InternalICs  ExternalResetVariant=Disabled  TRSumVariant=Passthrough  SumFdbkVariant=Disabled  SumVariant=Sum_PID  TsampFilterVariant=InternalTs  TsampNgainVariant=Passthrough  TsampIntegralVariant=Passthrough
  PID Controller2 : simulink/Continuous/PID Controller  Controller=PID  Form=Parallel  TimeDomain=Continuous-time  UseExternalTs=off  SampleTime=-1  IntegratorMethod=Forward Euler  FilterMethod=Forward Euler  ControllerParametersSource=internal  P=.01  I=1  D=0  UseFilter=on  N=100  TunerSelectOption=Transfer Function Based (PID Tuner App)  InitialConditionSource=internal  InitialConditionForIntegrator=0  InitialConditionForFilter=0  DifferentiatorICPrevScaledInput=0  ExternalReset=none  TrackingMode=off  Kt=1  LimitOutput=off  UpperSaturationLimit=inf  LowerSaturationLimit=-inf  LinearizeAsGain=on  AntiWindupMode=none  Kb=1  POutMin=[]  POutMax=[]  IOutMin=[]  IOutMax=[]  DOutMin=[]  DOutMax=[]  NOutMin=[]  NOutMax=[]  SumOutMin=[]  SumOutMax=[]  SaturationOutMin=[]  SaturationOutMax=[]  PParamMin=[]  PParamMax=[]  IParamMin=[]  IParamMax=[]  DParamMin=[]  DParamMax=[]  NParamMin=[]  NParamMax=[]  KbParamMin=[]  KbParamMax=[]  KtParamMin=[]  KtParamMax=[]  KbOutMin=[]  KbOutMax=[]  KtOutMin=[]  KtOutMax=[]  IntegratorOutMin=[]  IntegratorOutMax=[]  FilterOutMin=[]  FilterOutMax=[]  SumI1OutMin=[]  SumI1OutMax=[]  SumI2OutMin=[]  SumI2OutMax=[]  SumI3OutMin=[]  SumI3OutMax=[]  SumI4OutMin=[]  SumI4OutMax=[]  SumDOutMin=[]  SumDOutMax=[]  DifferentiatorOutMin=[]  DifferentiatorOutMax=[]  FilterDiffOutCoefMin=[]  FilterDiffOutCoefMax=[]  ReciprocalOutMin=[]  ReciprocalOutMax=[]  SumDenOutMin=[]  SumDenOutMax=[]  SumNumOutMin=[]  SumNumOutMax=[]  DivideOutMin=[]  DivideOutMax=[]  UdiffTsProdOutMin=[]  UdiffTsProdOutMax=[]  NTsProdOutMin=[]  NTsProdOutMax=[]  UintegralTsProdOutMin=[]  UintegralTsProdOutMax=[]  UngainTsProdOutMin=[]  UngainTsProdOutMax=[]  IntegratorContinuousStateAttributes=''  IntegratorStateMustResolveToSignalObject=off  IntegratorRTWStateStorageClass=Auto  FilterContinuousStateAttributes=''  FilterStateMustResolveToSignalObject=off  FilterRTWStateStorageClass=Auto  ParallelPVariant=InternalParameters  IdealPVariant=Disabled  IVariant=InternalParameters  DVariant=InternalParameters  IntegratorVariant=Continuous  SatVariant=Disabled  AWVariant=Passthrough  PCopyVariant=Disabled  TRVariant=Disabled  FdbkBlocksVariant=Forward  IdealPFdbkVariant=Disabled  SatFdbkVariant=Disabled  DerivativeFilterVariant=ContFilter  NVariant=InternalParameters  NCopyVariant=Disabled  FilterICVariant=InternalICsFilter  IntegratorICVariant=InternalICs  ExternalResetVariant=Disabled  TRSumVariant=Passthrough  SumFdbkVariant=Disabled  SumVariant=Sum_PID  TsampFilterVariant=InternalTs  TsampNgainVariant=Passthrough  TsampIntegralVariant=Passthrough
  Scope : Scope
  Scope1 : Scope
  Scope2 : Scope
  Sum : Sum  Inputs=|+-+
  Sum1 : Sum  Inputs=-+
  Sum2 : Sum  Inputs=-+
  Sum3 : Sum  Inputs=|+++
  Sum5 : Sum  Inputs=|+-
  Terminator{,1..3} (4 alike) : Terminator
  V_bc to V_dq0 : powerlib_meascontrol/Transformations/abc to dq0  Alignment=90 degrees behind phase A axis
  Vdc_ref : Constant  Value=600  VectorParams1D=off  SampleTime=-1
  abc to Alpha-Beta-Zero1 : powerlib_meascontrol/Transformations/abc to Alpha-Beta-Zero
  dq0 to abc : powerlib_meascontrol/Transformations/dq0 to abc  Alignment=90 degrees behind phase A axis
  iabc to idq0 : powerlib_meascontrol/Transformations/abc to dq0  Alignment=90 degrees behind phase A axis
  wLf : Gain  Gain=2*3.14*50*208.437e-6
  wLf1 : Gain  Gain=2*3.14*50*208.437e-6
  M : Outport
  wires:
  Vabc/1 -> abc to Alpha-Beta-Zero1/1, V_bc to V_dq0/1
  MSOGI_FLL1/2(Vβ) -> Terminator1/1
  V_bc to V_dq0/1 -> Demux1/1
  Demux1/3 -> Terminator2/1
  Demux2/3 -> Terminator/1
  iabc to idq0/1 -> Demux2/1
  Iabc/1 -> iabc to idq0/1
  Demux1/1 -> Sum/1
  wLf/1 -> Sum/2
  Demux2/2 -> Sum5/2, wLf/1
  Sum1/1 -> PID Controller/1
  Vdc/1 -> Sum1/1
  PID Controller/1 -> Sum2/2
  Demux2/1 -> wLf1/1, Sum2/1
  Vdc_ref/1 -> Sum1/2
  Sum2/1 -> PID Controller1/1
  PID Controller1/1 -> Sum/3
  Mux/1 -> dq0 to abc/1
  MSOGI_FLL1/3(ώt) -> V_bc to V_dq0/2, iabc to idq0/2, dq0 to abc/2, Scope2/1
  Sum/1 -> Mux/1
  Sum3/1 -> Mux/2
  Constant/1 -> Mux/3
  PID Controller2/1 -> Sum3/3
  Demux1/2 -> Sum3/1
  wLf1/1 -> Sum3/2
  Sum5/1 -> PID Controller2/1
  Iq_ref/1 -> Sum5/1
  abc to Alpha-Beta-Zero1/1 -> Gain1/1
  Gain1/1 -> Scope/1, MSOGI_FLL1/1(Vαβ0)
  MSOGI_FLL1/1(Vα) -> Terminator3/1
  dq0 to abc/1 -> Scope1/1, M/1

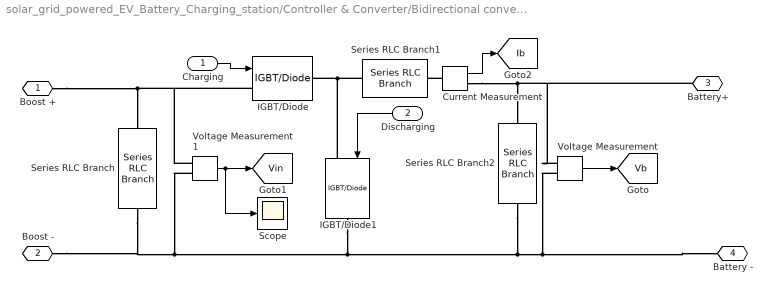
== system solar_grid_powered_EV_Battery_Charging_station/Controller & Converter/Bidirectional converter with battery controller/Bi-directional Converter ==
  Charging : Inport
  Discharging : Inport  Port=2
  Current Measurement : powerlib/Measurements/Current Measurement  PhasorSimulation=off  OutputType=Complex  PSBequivalent=0
  IGBT/Diode : powerlib/Power Electronics/IGBT//Diode  Ron=1e-3  Rs=1e5  Cs=inf  Measurements=off
  IGBT/Diode1 : powerlib/Power Electronics/IGBT//Diode  Ron=1e-3  Rs=1e5  Cs=inf  Measurements=off
  Scope : Scope
  Series RLC Branch : powerlib/Elements/Series RLC Branch  LConnTagsString=__new0  RConnTagsString=__new0  BranchType=RC  Resistance=.0001  Inductance=1e-3  SetiL0=off  InitialCurrent=0  Capacitance=3000e-6  Setx0=off  InitialVoltage=0  Measurements=None
  Series RLC Branch1 : powerlib/Elements/Series RLC Branch  LConnTagsString=__new0  RConnTagsString=__new0  BranchType=L  Resistance=1  Inductance=200e-3  SetiL0=off  InitialCurrent=0  Capacitance=1e-6  Setx0=off  InitialVoltage=0  Measurements=None
  Series RLC Branch2 : powerlib/Elements/Series RLC Branch  LConnTagsString=__new0  RConnTagsString=__new0  BranchType=C  Resistance=.0001  Inductance=1e-3  SetiL0=off  InitialCurrent=0  Capacitance=30e-6  Setx0=off  InitialVoltage=0  Measurements=None
  Voltage Measurement : powerlib/Measurements/Voltage Measurement  PhasorSimulation=off  OutputType=Complex  PSBequivalent=0
  Voltage Measurement1 : powerlib/Measurements/Voltage Measurement  PhasorSimulation=off  OutputType=Complex  PSBequivalent=0
  Boost + : PMIOPort  Side=Left
  Boost - : PMIOPort  Port=2  Side=Left
  Battery+ : PMIOPort  Port=3  Side=Right
  Battery - : PMIOPort  Port=4  Side=Right
  tag scope: Ib=global, Vb=global, Vin=global
  wires:
  Current Measurement/1 -> [Ib]
  Voltage Measurement/1 -> [Vb]
  Voltage Measurement1/1 -> Scope/1, [Vin]
  Charging/1 -> IGBT/Diode/1
  Discharging/1 -> IGBT/Diode1/1
  connections:
  Current Measurement/RConn1 -- Battery+/RConn1 -- Voltage Measurement/LConn1 -- Series RLC Branch2/LConn1
  IGBT/Diode1/LConn1 -- Series RLC Branch1/LConn1 -- IGBT/Diode/RConn1
  Current Measurement/LConn1 -- Series RLC Branch1/RConn1
  IGBT/Diode/LConn1 -- Voltage Measurement1/LConn1 -- Boost +/RConn1 -- Series RLC Branch/LConn1
  Voltage Measurement1/LConn2 -- Series RLC Branch/RConn1 -- Boost -/RConn1 -- IGBT/Diode1/RConn1 -- Series RLC Branch2/RConn1 -- Voltage Measurement/LConn2 -- Battery -/RConn1

== system solar_grid_powered_EV_Battery_Charging_station/Controller & Converter/Bidirectional converter with battery controller/controller ==
  note: Discharging
  note: Charging
  Vin : Inport
  Ib : Inport  Port=2
  Vb : Inport  Port=3
  CONTROL : Inport  Port=4
  Constant : Constant  Value=0
  Constant1 : Constant  Value=0
  Duty Cycle : Subsystem
  Duty Cycle1 : Subsystem
  Switch : Switch  Criteria=u2 > Threshold
  Switch1 : Switch  Criteria=u2 > Threshold
  pwm : Subsystem
  pwm1 : Subsystem
  pwm_discharging : Outport
  pwm_charging : Outport  Port=2
  wires:
  Ib/1 -> Duty Cycle1/2(Ib)
  Vin/1 -> Duty Cycle1/1(Vin)
  Duty Cycle/1(D) -> pwm/1(Duty)
  Duty Cycle1/1(D) -> pwm1/1(Duty)
  Vb/1 -> Duty Cycle/1(Vb)
  CONTROL/1 -> Switch/2, Switch1/2
  pwm/1(pwm) -> Switch/3
  Switch/1 -> pwm_charging/1
  Constant/1 -> Switch/1
  pwm1/1(pwm) -> Switch1/1
  Switch1/1 -> pwm_discharging/1
  Constant1/1 -> Switch1/3

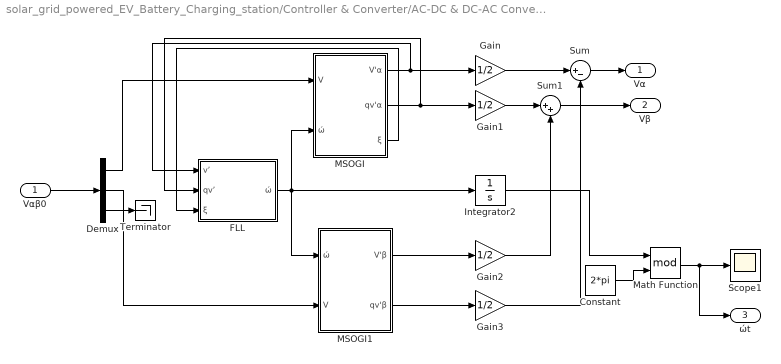
== system solar_grid_powered_EV_Battery_Charging_station/Controller & Converter/AC-DC & DC-AC Converter/controller1/MSOGI_FLL1 ==
  Vαβ0 : Inport
  Constant : Constant  Value=2*pi
  Demux : Demux  Outputs=3
  FLL : Subsystem
  Gain{,1..3} (4 alike) : Gain  Gain=1/2
  Integrator2 : Integrator
  MSOGI : Subsystem
  MSOGI1 : Subsystem
  Math Function : Math  Operator=mod  SaturateOnIntegerOverflow=on
  Scope1 : Scope
  Sum : Sum  Inputs=|+-
  Sum1 : Sum  Inputs=|++
  Terminator : Terminator
  Vα : Outport
  Vβ : Outport  Port=2
  ώt : Outport  Port=3
  wires:
  MSOGI/3(ξ) -> FLL/3(ξ)
  Gain1/1 -> Sum1/1
  MSOGI/1(V'α) -> FLL/1(v’), Gain/1
  FLL/1(ώ) -> MSOGI/2(ώ), Integrator2/1, MSOGI1/1(ώ)
  MSOGI/2(qv'α) -> FLL/2(qv’), Gain1/1
  Gain/1 -> Sum/1
  Demux/3 -> Terminator/1
  MSOGI1/1(V'β) -> Gain2/1
  Demux/1 -> MSOGI/1(V)
  MSOGI1/2(qv'β) -> Gain3/1
  Gain3/1 -> Sum/2
  Demux/2 -> MSOGI1/2(V)
  Vαβ0/1 -> Demux/1
  Gain2/1 -> Sum1/2
  Sum/1 -> Vα/1
  Sum1/1 -> Vβ/1
  Integrator2/1 -> Math Function/1
  Math Function/1 -> ώt/1, Scope1/1
  Constant/1 -> Math Function/2
